simulink model "observersimualtion"  (R2015a)
settings: Solver=ode45  StartTime=0.0  StopTime=20  RelTol=1e-6
values from neighbouring files (symbols this model uses):
  d0 = 1.5897e-3    (= 0.0015897)    [initialise.m]
  d1 = 1.773e-6    (= 1.773e-06)    [initialise.m]
  g = 9.81    [initialise.m]
  J0 = 1.4316e-4    (= 0.00014316)    [initialise.m]
  J1 = 2.078867e-4    (= 0.0002078867)    [initialise.m]
  Kf = 0.05722    [initialise.m]
  Kg = 13/18    (= 0.722222222222)    [initialise.m]
  Kt = 0.05722    [initialise.m]
  L = place(sys_d.a',[1 0 0 0;0 0 1 0]',P)'    [BuildController.m]
  L0 = 0.09    [initialise.m]
  L1 = 0.225    [initialise.m]
  m1 = 0.009    [initialise.m]
  Ra = 17    [initialise.m]
undefined symbols (not defined in the file): sys_d
settings Model: Creator=Alvin  LastModifiedBy=Alvin
settings SolverCC: AlgebraicLoopSolver=LineSearch
settings DataIOCC: SaveState=on

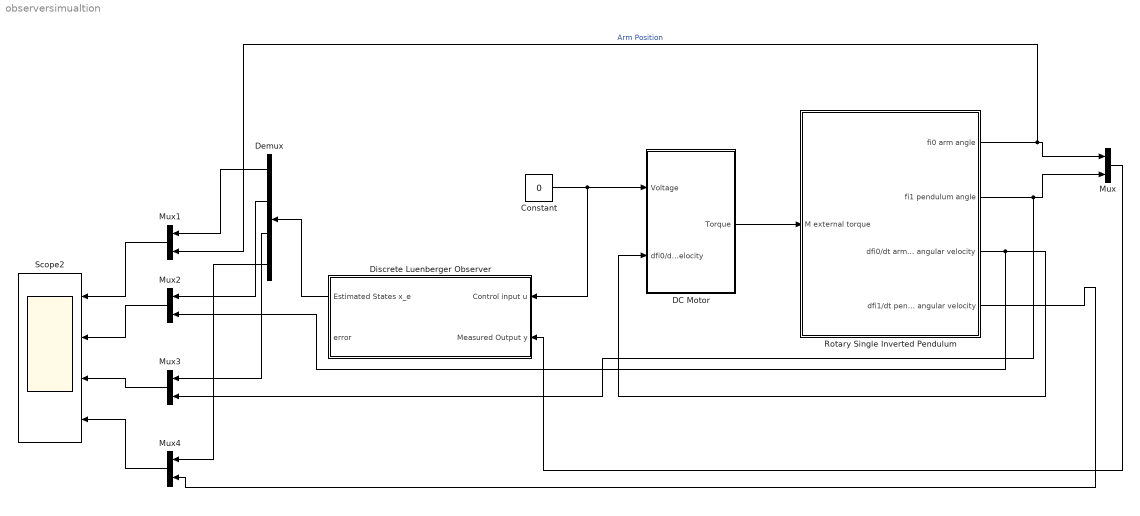
== system observersimualtion ==
  Constant : Constant  Value=0
  DC Motor : Subsystem
  Demux : Demux
  Discrete Luenberger Observer : Subsystem  mask{A=sys_d.a, B=sys_d.b, C=[1 0 0 0; 0 0 1 0], L=L, SampleTime=0.025}
      mask prompts: A "Discretized state matrix A:"; B "Discretized input matrix B:"; C "Output matrix C:"; L "Discretized observer gain matrix L:"; SampleTime "Sample Time (-1 for inherited):"
      mask TypeOptions A: A/Gain
      mask TypeOptions B: B/Gain
      mask TypeOptions C: C/Gain
      mask TypeOptions L: L/Gain
      mask TypeOptions SampleTime:
      | Zero-Order
      | Hold1/SampleTime
      mask DialogControl DescTextVar Prompt: The Luenberger Observer block implements a discrete time Luenberger Observer. Use this block to estimate the states of an observable system using:  The discrete inputs and outputs of the system. A discrete state-space representation of the system. The Luenberger Observer is also sometimes referred to as a state observer or simply an observer.  You can control multi-input, multi-output systems by passing the output state vector of this block to a State Feedback Controller block.
  Mux{,1..4} (5 alike) : Mux  Inputs=2
  Rotary Single Inverted Pendulum : Subsystem  mask{fi1=0.00001}
      mask prompts: fi1 "Pendulum Position Initial Condition"
      mask TypeOptions fi1: Pendulum/Constant/Value
  Scope2 : Scope  NumInputPorts=4
      settings: YMin=-5~-5~-5~-5  YMax=5~5~5~5  SaveName=ScopeData_obs
  wires:
  DC Motor/1(Torque) -> Rotary Single Inverted Pendulum/1(M external torque)
  Rotary Single Inverted Pendulum/3(dfi0/dt arm angular velocity) -> Mux2/2, DC Motor/2(dfi0/dt Arm Angular Velocity)
  Constant/1 -> Discrete Luenberger Observer/1(Control input u), DC Motor/1(Voltage)
  Rotary Single Inverted Pendulum/1(fi0 arm angle) -> Mux1/2, Mux/1  "Arm Position"
  Rotary Single Inverted Pendulum/2(fi1 pendulum angle) -> Mux3/2, Mux/2
  Mux/1 -> Discrete Luenberger Observer/2(Measured Output y)
  Discrete Luenberger Observer/1(Estimated States x_e) -> Demux/1
  Rotary Single Inverted Pendulum/4(dfi1/dt pendulum angular velocity) -> Mux4/2
  Demux/1 -> Mux1/1
  Demux/2 -> Mux2/1
  Demux/3 -> Mux3/1
  Demux/4 -> Mux4/1
  Mux1/1 -> Scope2/1
  Mux2/1 -> Scope2/2
  Mux3/1 -> Scope2/3
  Mux4/1 -> Scope2/4

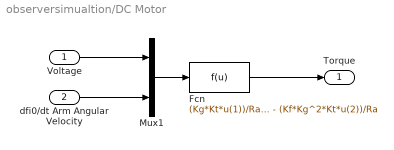
== system observersimualtion/DC Motor ==
  Voltage : Inport
  dfi0/dt Arm Angular Velocity : Inport  Port=2
  Fcn : Fcn  Expr=(Kg*Kt*u(1))/Ra - (Kf*Kg^2*Kt*u(2))/Ra
  Mux1 : Mux  Inputs=2
  Torque : Outport
  wires:
  dfi0/dt Arm Angular Velocity/1 -> Mux1/2
  Mux1/1 -> Fcn/1
  Fcn/1 -> Torque/1
  Voltage/1 -> Mux1/1

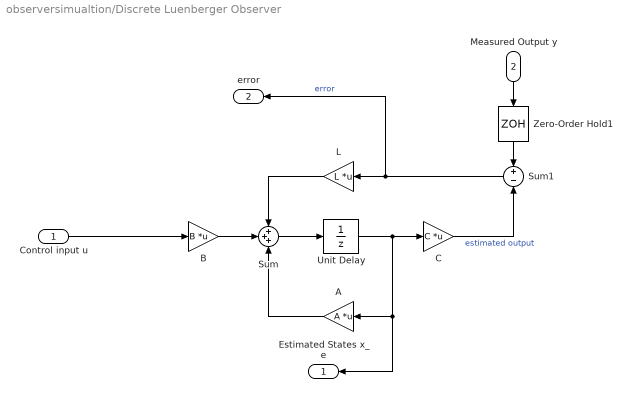
== system observersimualtion/Discrete Luenberger Observer ==
  Control input u : Inport
  Measured Output y : Inport  Port=2
  A : Gain  Gain=A  Multiplication=Matrix(K*u)
  B : Gain  Gain=B  Multiplication=Matrix(K*u)
  C : Gain  Gain=C  Multiplication=Matrix(K*u)
  L : Gain  Gain=L  Multiplication=Matrix(K*u)
  Sum : Sum  Inputs=+++
  Sum1 : Sum  Inputs=+-
  Unit Delay : UnitDelay  SampleTime=-1
  Zero-Order Hold1 : ZeroOrderHold  SampleTime=SampleTime
  Estimated States x_e : Outport
  error : Outport  Port=2
  wires:
  Sum1/1 -> error/1, L/1  "error"
  A/1 -> Sum/3
  B/1 -> Sum/2
  C/1 -> Sum1/2  "estimated output"
  L/1 -> Sum/1
  Unit Delay/1 -> Estimated States x_e/1, A/1, C/1
  Sum/1 -> Unit Delay/1
  Control input u/1 -> B/1
  Measured Output y/1 -> Zero-Order Hold1/1
  Zero-Order Hold1/1 -> Sum1/1

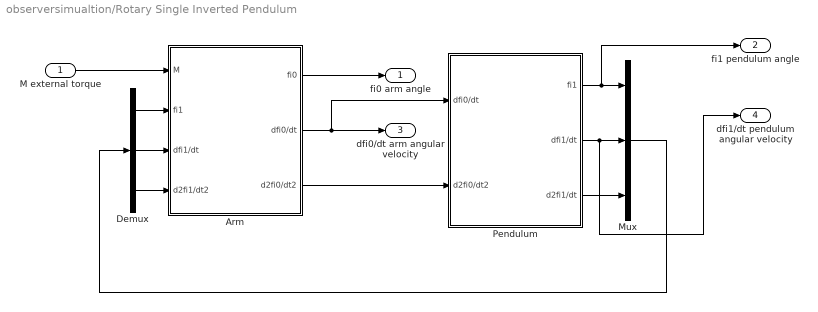
== system observersimualtion/Rotary Single Inverted Pendulum ==
  M external torque : Inport
  Arm : Subsystem
  Demux : Demux  Outputs=3
  Mux : Mux  Inputs=3
  Pendulum : Subsystem
  fi0 arm angle : Outport
  fi1 pendulum angle : Outport  Port=2
  dfi0/dt arm angular velocity : Outport  Port=3
  dfi1/dt pendulum angular velocity : Outport  Port=4
  wires:
  Pendulum/1(fi1) -> fi1 pendulum angle/1, Mux/1
  Pendulum/2(dfi1/dt) -> dfi1/dt pendulum angular velocity/1, Mux/2
  Mux/1 -> Demux/1
  Demux/1 -> Arm/2(fi1)
  Demux/2 -> Arm/3(dfi1/dt)
  Demux/3 -> Arm/4(d2fi1/dt2)
  M external torque/1 -> Arm/1(M)
  Pendulum/3(d2fi1/dt) -> Mux/3
  Arm/3(d2fi0/dt2) -> Pendulum/2(d2fi0/dt2)
  Arm/1(fi0) -> fi0 arm angle/1
  Arm/2(dfi0/dt) -> dfi0/dt arm angular velocity/1, Pendulum/1(dfi0/dt)

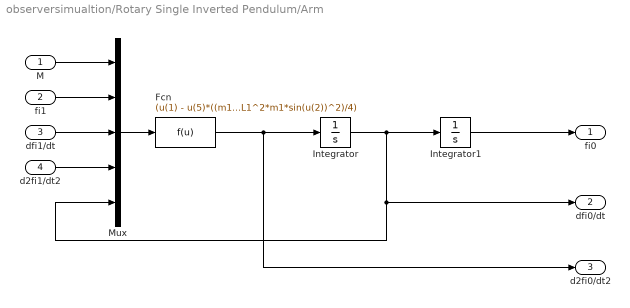
== system observersimualtion/Rotary Single Inverted Pendulum/Arm ==
  M : Inport
  fi1 : Inport  Port=2
  dfi1/dt : Inport  Port=3
  d2fi1/dt2 : Inport  Port=4
  Fcn : Fcn  Expr=(u(1) - u(5)*((m1*u(3)*sin(2*u(2))*L1^2)/4 + d0) + (L0*L1*m1*u(3)^2*sin(u(2)))/2 - (L0*L1*m1*u(4)*cos(u(2)))/2)/(J0 + L0^2*m1 + (L1^2*m1*sin(u(2))^2)/4)
  Integrator : Integrator
  Integrator1 : Integrator
  Mux : Mux  Inputs=5
  fi0 : Outport
  dfi0/dt : Outport  Port=2
  d2fi0/dt2 : Outport  Port=3
  wires:
  Mux/1 -> Fcn/1
  Fcn/1 -> d2fi0/dt2/1, Integrator/1
  Integrator/1 -> dfi0/dt/1, Mux/5, Integrator1/1
  Integrator1/1 -> fi0/1
  fi1/1 -> Mux/2
  dfi1/dt/1 -> Mux/3
  M/1 -> Mux/1
  d2fi1/dt2/1 -> Mux/4

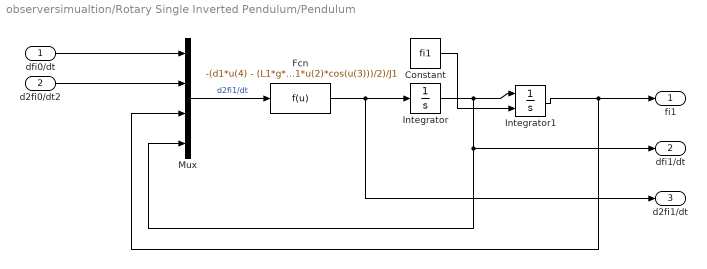
== system observersimualtion/Rotary Single Inverted Pendulum/Pendulum ==
  dfi0/dt : Inport
  d2fi0/dt2 : Inport  Port=2
  Constant : Constant  Value=fi1
  Fcn : Fcn  Expr=-(d1*u(4) - (L1*g*m1*sin(u(3)))/2 - (L1^2*m1*u(1)^2*sin(2*u(3)))/8 + (L0*L1*m1*u(2)*cos(u(3)))/2)/J1
  Integrator : Integrator
  Integrator1 : Integrator  InitialConditionSource=external
  Mux : Mux
  fi1 : Outport
  dfi1/dt : Outport  Port=2
  d2fi1/dt : Outport  Port=3
  wires:
  Integrator1/1 -> fi1/1, Mux/3
  Fcn/1 -> d2fi1/dt/1, Integrator/1
  Mux/1 -> Fcn/1  "d2fi1/dt"
  Integrator/1 -> dfi1/dt/1, Mux/4, Integrator1/1
  dfi0/dt/1 -> Mux/1
  d2fi0/dt2/1 -> Mux/2
  Constant/1 -> Integrator1/2
